simulink model "control_PV"  (R2019b)
settings: Solver=VariableStepAuto  StartTime=0.0  StopTime=500  RelTol=1e-3
undefined symbols (not defined in the file): sgn
libraries: simulink x1
settings Model: Creator=Alejandro  LastModifiedBy=Alejandro
settings SolverCC: ZeroCrossAlgorithm=Adaptive
settings DebuggingCC: IgnoredZcDiagnostic=none

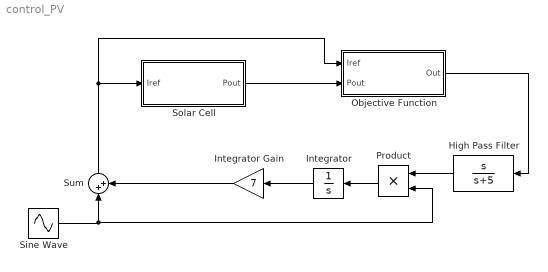
== system control_PV ==
  High Pass Filter : TransferFcn  Numerator=[1 0]  Denominator=[1 5]
  Integrator : Integrator
  Integrator Gain : Gain  Gain=7
  Objective Function : Subsystem  TreatAsAtomicUnit=on
  Product : Product
  Sine Wave : Sin  Amplitude=0.05  Frequency=5*2*pi  SampleTime=0
  Solar Cell : Subsystem
  Sum : Sum  Inputs=|++
  wires:
  High Pass Filter/1 -> Product/1
  Sine Wave/1 -> Product/2, Sum/1
  Product/1 -> Integrator/1
  Integrator/1 -> Integrator Gain/1
  Integrator Gain/1 -> Sum/2
  Objective Function/1(Out) -> High Pass Filter/1
  Solar Cell/1("Pout ") -> Objective Function/2(Pout)
  Sum/1 -> Objective Function/1(Iref), Solar Cell/1("Iref ")

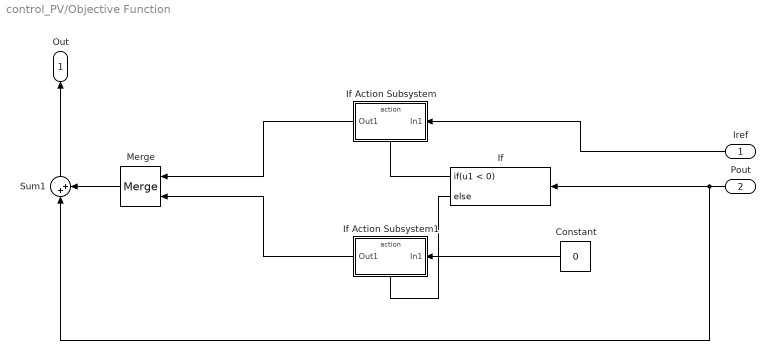
== system control_PV/Objective Function ==
  Iref : Inport
  Pout : Inport  Port=2
  Constant : Constant  Value=0
  If : If  IfExpression=u1 < 0
  If Action Subsystem : Subsystem  TreatAsAtomicUnit=on
  If Action Subsystem1 : Subsystem  TreatAsAtomicUnit=on
  Merge : Merge
  Sum1 : Sum  Inputs=|++
  Out : Outport
  wires:
  If Action Subsystem1/1(Out1) -> Merge/2
  Constant/1 -> If Action Subsystem1/1(In1)
  If/2 -> If Action Subsystem1/Action
  If Action Subsystem/1(Out1) -> Merge/1
  If/1 -> If Action Subsystem/Action
  Iref/1 -> If Action Subsystem/1(In1)
  Merge/1 -> Sum1/2
  Pout/1 -> Sum1/1, If/1
  Sum1/1 -> Out/1

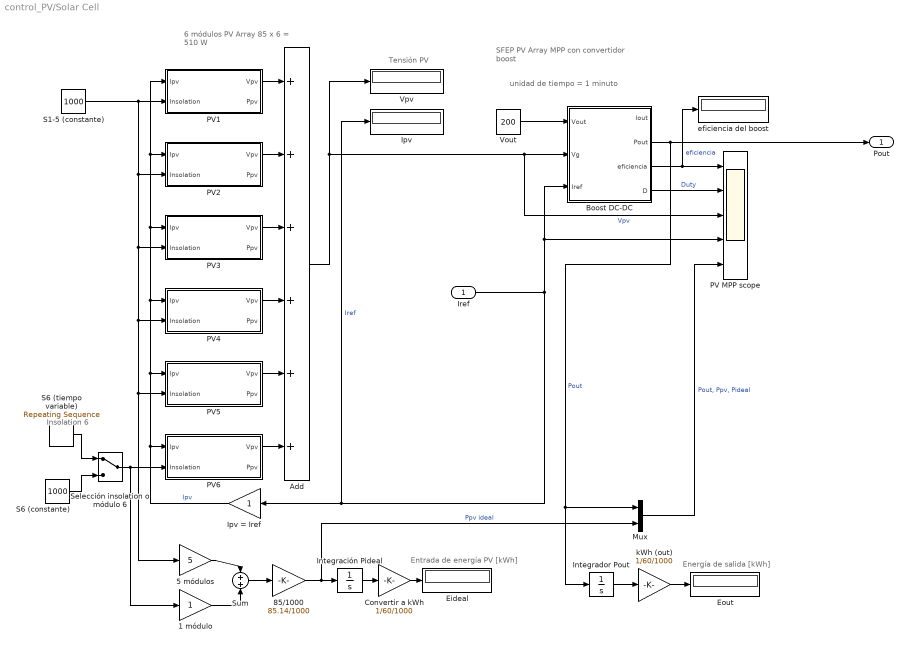
== system control_PV/Solar Cell ==
  note: 6 módulos PV Array
      | 85 x 6 = 510 W
  note: Insolation 6
  note: unidad de tiempo = 1 minuto
  note: SFEP
      | PV Array MPP con convertidor boost
  note: Entrada de energía PV [kWh]
  note: Energía de salida [kWh]
  note: Tensión PV
  "Iref " : Inport
  1 módulo : Gain
  5 módulos : Gain  Gain=5
  85/1000 : Gain  Gain=85.14/1000
  Add : Sum  Inputs=++++++
  Boost DC-DC : Subsystem  mask{RL=0.5, Isw=0.03}
      mask prompts: RL "Resistencia de pérdidas de conducción RL"; Isw "Pérdidas de conmutación Isw"
      mask help: Modelo promediado del boost con corriente de referencia como variable de control. El modelo incluye las pérdidas por conducción en serie con la entrada y la corriente de pérdidas por conmutación en paralelo con la salida.
      mask Display:
      | text(0.5,0.9,'Boost','horizontalAlignment', 'center');
      | text(0.5,0.8,'DC-DC','horizontalAlignment', 'center');
      | text(0.5,0.7,'(control Iref)','horizontalAlignment', 'center');
      | text(0.5,0.6,'promediado','horizontalAlignment', 'center');
  Convertir a kWh : Gain  Gain=1/60/1000
  Eideal : Display
  Eout : Display
  Integración Pideal : Integrator
  Integrador Pout : Integrator
  Ipv : Display
  Ipv = Iref : Gain
  Mux : Mux  Inputs=3
  PV MPP scope : Scope  NumInputPorts=5
  PV1 : Subsystem  mask{Isc=5.45, Voc=22.2, Ir=4.95, Vr=17.2}
      mask prompts: Isc "Corriente de cortocircuito"; Voc "Tensión en circuito abierto"; Ir "Corriente a Pmax"; Vr "Tensión a Pmáx"
      mask help: Modelo de módulo PV. Este modelo tiene entrada de Vpv para realizar conexión en paralelo.
      mask init:
      | % cálculo de PV parámetros
      | % limitación: constante de temperatura
      | Ns = round(Voc/0.61); % por defecto, número de células en serie
      | Vt = 26e-3; % tensión de temperatura
      | G = Isc/1000; % Ganancia de irradiación en función del cortocircuito
      | Vmpc = Vr/Ns; % tensión de celda a Pmáx
      | Vocc = Voc/Ns; % tensión de celda a circuito abierto
      | Rmpp = Vmpc/Ir; % resistencia de carga 
      | %
      | Rp = 100*Vocc/Isc; % valor inicial de Rp
      | Vdm = Vocc; % valor inicial para Vm
      | %
      | % solución iterativa para el modelo: Io, Rs, Rp
      | for i=1:10
      | %
      |  Idm = Isc - Ir - Vdm/Rp; % pn-junction (diodo) corriente a MPP
      |  Io = (Isc-Vocc/Rp)/(exp(Vocc/Vt)-1); % pn-junction corriente inversa de saturación
      |  Vdm = Vt*log(Idm/Io+1); % pn-junction (diodo) tensión a MPP
      |  Rs = (Vdm-Vmpc)/Ir; % resistencia serie
      |  Rd = (Rmpp - Rs)*Rp/(Rp-Rmpp+Rs); % resistencia incremental del diodo  a MPP
      |  Idm = Vt/Rd; % corriente del diodo a MPP basado en resistencia incremental
      |  Rp = Vdm/(Isc-Ir-Idm); % resistencia paralelo
      | %
      | end
      | %
      mask Display:
      | plot([0.3 0.4],[0.4 0.8]);
      | plot([0.4 0.5],[0.4 0.8]);
      | plot([0.5 0.6],[0.4 0.8]);
      | plot([0.6 0.7],[0.4 0.8]);
      | plot([0.3 0.6],[0.4 0.4]);
      | plot([0.325 0.625],[0.5 0.5]);
      | plot([0.35 0.65],[0.6 0.6]);
      | plot([0.375 0.675],[0.7 0.7]);
      | plot([0.4 0.7],[0.8 0.8]);
      | text(0.5,0.9,'Módulo PV','horizontalAlignment', 'center');
  PV2 : Subsystem  mask{Isc=5.45, Voc=22.2, Ir=4.95, Vr=17.2}
      mask prompts: Isc "Corriente de cortocircuito"; Voc "Tensión en circuito abierto"; Ir "Corriente a Pmax"; Vr "Tensión a Pmáx"
      mask help: Modelo de módulo PV. Este modelo tiene entrada de Vpv para realizar conexión en paralelo.
      mask init: same as control_PV/Solar Cell/PV1
      mask Display:
      | plot([0.3 0.4],[0.4 0.8]);
      | plot([0.4 0.5],[0.4 0.8]);
      | plot([0.5 0.6],[0.4 0.8]);
      | plot([0.6 0.7],[0.4 0.8]);
      | plot([0.3 0.6],[0.4 0.4]);
      | plot([0.325 0.625],[0.5 0.5]);
      | plot([0.35 0.65],[0.6 0.6]);
      | plot([0.375 0.675],[0.7 0.7]);
      | plot([0.4 0.7],[0.8 0.8]);
      | text(0.5,0.9,'Módulo PV','horizontalAlignment', 'center');
  PV3 : Subsystem  mask{Isc=5.45, Voc=22.2, Ir=4.95, Vr=17.2}
      mask prompts: Isc "Corriente de cortocircuito"; Voc "Tensión en circuito abierto"; Ir "Corriente a Pmax"; Vr "Tensión a Pmáx"
      mask help: Modelo de módulo PV. Este modelo tiene entrada de Vpv para realizar conexión en paralelo.
      mask init: same as control_PV/Solar Cell/PV1
      mask Display:
      | plot([0.3 0.4],[0.4 0.8]);
      | plot([0.4 0.5],[0.4 0.8]);
      | plot([0.5 0.6],[0.4 0.8]);
      | plot([0.6 0.7],[0.4 0.8]);
      | plot([0.3 0.6],[0.4 0.4]);
      | plot([0.325 0.625],[0.5 0.5]);
      | plot([0.35 0.65],[0.6 0.6]);
      | plot([0.375 0.675],[0.7 0.7]);
      | plot([0.4 0.7],[0.8 0.8]);
      | text(0.5,0.9,'Módulo PV','horizontalAlignment', 'center');
  PV4 : Subsystem  mask{Isc=5.45, Voc=22.2, Ir=4.95, Vr=17.2}
      mask prompts: Isc "Corriente de cortocircuito"; Voc "Tensión en circuito abierto"; Ir "Corriente a Pmax"; Vr "Tensión a Pmáx"
      mask help: Modelo de módulo PV. Este modelo tiene entrada de Vpv para realizar conexión en paralelo.
      mask init: same as control_PV/Solar Cell/PV1
      mask Display:
      | plot([0.3 0.4],[0.4 0.8]);
      | plot([0.4 0.5],[0.4 0.8]);
      | plot([0.5 0.6],[0.4 0.8]);
      | plot([0.6 0.7],[0.4 0.8]);
      | plot([0.3 0.6],[0.4 0.4]);
      | plot([0.325 0.625],[0.5 0.5]);
      | plot([0.35 0.65],[0.6 0.6]);
      | plot([0.375 0.675],[0.7 0.7]);
      | plot([0.4 0.7],[0.8 0.8]);
      | text(0.5,0.9,'Módulo PV','horizontalAlignment', 'center');
  PV5 : Subsystem  mask{Isc=5.45, Voc=22.2, Ir=4.95, Vr=17.2}
      mask prompts: Isc "Corriente de cortocircuito"; Voc "Tensión en circuito abierto"; Ir "Corriente a Pmax"; Vr "Tensión a Pmáx"
      mask help: Modelo de módulo PV. Este modelo tiene entrada de Vpv para realizar conexión en paralelo.
      mask init: same as control_PV/Solar Cell/PV1
      mask Display:
      | plot([0.3 0.4],[0.4 0.8]);
      | plot([0.4 0.5],[0.4 0.8]);
      | plot([0.5 0.6],[0.4 0.8]);
      | plot([0.6 0.7],[0.4 0.8]);
      | plot([0.3 0.6],[0.4 0.4]);
      | plot([0.325 0.625],[0.5 0.5]);
      | plot([0.35 0.65],[0.6 0.6]);
      | plot([0.375 0.675],[0.7 0.7]);
      | plot([0.4 0.7],[0.8 0.8]);
      | text(0.5,0.9,'Módulo PV','horizontalAlignment', 'center');
  PV6 : Subsystem  mask{Isc=5.45, Voc=22.2, Ir=4.95, Vr=17.2}
      mask prompts: Isc "Corriente de cortocircuito"; Voc "Tensión en circuito abierto"; Ir "Corriente a Pmax"; Vr "Tensión a Pmáx"
      mask help: Modelo de módulo PV. Este modelo tiene entrada de Vpv para realizar conexión en paralelo.
      mask init: same as control_PV/Solar Cell/PV1
      mask Display:
      | plot([0.3 0.4],[0.4 0.8]);
      | plot([0.4 0.5],[0.4 0.8]);
      | plot([0.5 0.6],[0.4 0.8]);
      | plot([0.6 0.7],[0.4 0.8]);
      | plot([0.3 0.6],[0.4 0.4]);
      | plot([0.325 0.625],[0.5 0.5]);
      | plot([0.35 0.65],[0.6 0.6]);
      | plot([0.375 0.675],[0.7 0.7]);
      | plot([0.4 0.7],[0.8 0.8]);
      | text(0.5,0.9,'Módulo PV','horizontalAlignment', 'center');
  S1-5 (constante) : Constant  Value=1000
  S6 (tiempo variable) : simulink/Sources/Repeating Sequence  rep_seq_t=[0 1*60 2*60 3*60 4*60 5*60 6*60 7*60 8*60]  rep_seq_y=[0 400 850 950 0 950 850 400 0]
  S6 (constante) : Constant  Value=1000
  Selección insolation o módulo 6 : ManualSwitch
  Sum : Sum  Inputs=+|+
  Vout : Constant  Value=200
  Vpv : Display
  eficiencia del boost : Display
  kWh (out) : Gain  Gain=1/60/1000
  "Pout " : Outport
  wires:
  PV1/1(Vpv) -> Add/1
  Ipv = Iref/1 -> PV2/1(Ipv), PV1/1(Ipv), PV3/1(Ipv), PV4/1(Ipv), PV5/1(Ipv), PV6/1(Ipv)  "Ipv"
  PV2/1(Vpv) -> Add/2
  Boost DC-DC/2(Pout) -> "Pout "/1, Mux/1, Integrador Pout/1  "Pout"
  S6 (tiempo variable)/1 -> Selección insolation o módulo 6/1
  kWh (out)/1 -> Eout/1
  "Iref "/1 -> Ipv = Iref/1, Ipv/1, Boost DC-DC/3(Iref), PV MPP scope/4  "Iref"
  PV6/1(Vpv) -> Add/6
  Boost DC-DC/3(eficiencia) -> eficiencia del boost/1, PV MPP scope/1  "eficiencia"
  Selección insolation o módulo 6/1 -> 1 módulo/1, PV6/2(Insolation)
  Convertir a kWh/1 -> Eideal/1
  Integrador Pout/1 -> kWh (out)/1
  PV4/1(Vpv) -> Add/4
  Vout/1 -> Boost DC-DC/1(Vout)
  Add/1 -> Vpv/1, Boost DC-DC/2(Vg), PV MPP scope/3  "Vpv"
  Boost DC-DC/4(D) -> PV MPP scope/2  "Duty"
  5 módulos/1 -> Sum/1
  Sum/1 -> 85/1000/1
  PV3/1(Vpv) -> Add/3
  1 módulo/1 -> Sum/2
  85/1000/1 -> Integración Pideal/1, Mux/3  "Ppv ideal"
  Mux/1 -> PV MPP scope/5  "Pout, Ppv, Pideal"
  S1-5 (constante)/1 -> 5 módulos/1, PV5/2(Insolation), PV4/2(Insolation), PV3/2(Insolation), PV2/2(Insolation), PV1/2(Insolation)
  PV5/1(Vpv) -> Add/5
  S6 (constante)/1 -> Selección insolation o módulo 6/2
  Integración Pideal/1 -> Convertir a kWh/1

== system control_PV/Objective Function/If Action Subsystem ==
  In1 : Inport
  Action Port : ActionPort  ActionPortLabel=if(u1 < 0)
  Fcn : Fcn  Expr=-sgn(u)*u*5-6
  Out1 : Outport
  wires:
  In1/1 -> Fcn/1
  Fcn/1 -> Out1/1

== system control_PV/Objective Function/If Action Subsystem1 ==
  In1 : Inport
  Action Port : ActionPort  ActionPortLabel=else
  Out1 : Outport
  wires:
  In1/1 -> Out1/1

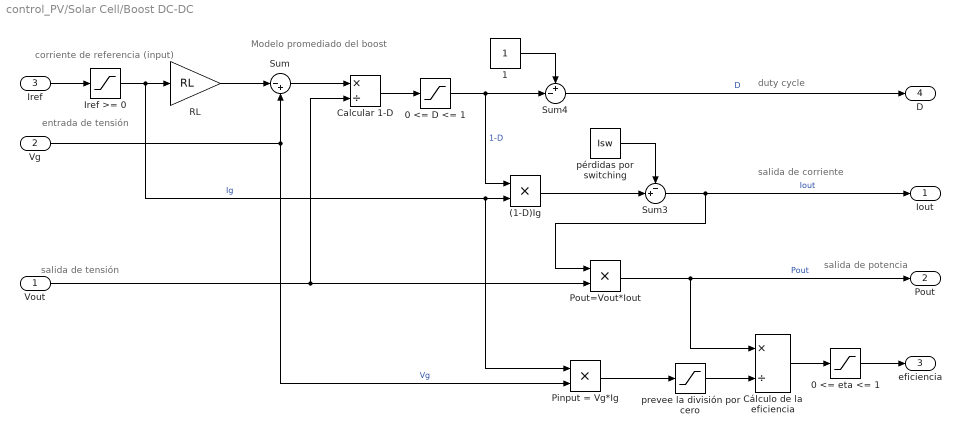
== system control_PV/Solar Cell/Boost DC-DC ==
  note: Modelo promediado del boost
  note: salida de corriente
  note: salida de tensión
  note: entrada de tensión
  note: corriente de
      | referencia (input)
  note: duty cycle
  note: salida de potencia
  Vout : Inport
  Vg : Inport  Port=2
  Iref : Inport  Port=3
  (1-D)Ig : Product  Inputs=**  RndMeth=Zero
  0 <= D <= 1 : Saturate  UpperLimit=1  LowerLimit=0
  0 <= eta <= 1 : Saturate  UpperLimit=1  LowerLimit=0
  1 : Constant
  Calcular 1-D : Product  Inputs=*/  RndMeth=Zero
  Cálculo de la eficiencia : Product  Inputs=*/  RndMeth=Zero
  Iref >= 0 : Saturate  UpperLimit=inf  LowerLimit=0
  Pinput = Vg*Ig : Product  Inputs=**  RndMeth=Zero
  Pout=Vout*Iout : Product  Inputs=**  RndMeth=Zero
  RL : Gain  Gain=RL
  Sum : Sum  Inputs=|-+
  Sum3 : Sum  Inputs=-+|
  Sum4 : Sum  Inputs=+-|
  prevee la división por cero : Saturate  UpperLimit=inf  LowerLimit=eps
  pérdidas por switching : Constant  Value=Isw
  Iout : Outport
  Pout : Outport  Port=2
  eficiencia : Outport  Port=3
  D : Outport  Port=4
  wires:
  Cálculo de la eficiencia/1 -> 0 <= eta <= 1/1
  Iref/1 -> Iref >= 0/1
  Vout/1 -> Pout=Vout*Iout/2, Calcular 1-D/2
  pérdidas por switching/1 -> Sum3/1
  Sum3/1 -> Iout/1, Pout=Vout*Iout/1  "Iout"
  Pout=Vout*Iout/1 -> Pout/1, Cálculo de la eficiencia/1  "Pout"
  0 <= eta <= 1/1 -> eficiencia/1
  Iref >= 0/1 -> RL/1, (1-D)Ig/2, Pinput = Vg*Ig/1  "Ig"
  RL/1 -> Sum/1
  Vg/1 -> Sum/2, Pinput = Vg*Ig/2  "Vg"
  Sum/1 -> Calcular 1-D/1
  Calcular 1-D/1 -> 0 <= D <= 1/1
  0 <= D <= 1/1 -> Sum4/2, (1-D)Ig/1  "1-D"
  1/1 -> Sum4/1
  Sum4/1 -> D/1  "D"
  (1-D)Ig/1 -> Sum3/2
  prevee la división por cero/1 -> Cálculo de la eficiencia/2
  Pinput = Vg*Ig/1 -> prevee la división por cero/1

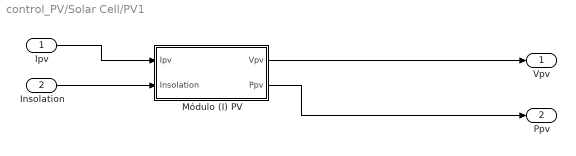
== system control_PV/Solar Cell/PV1 ==
  Ipv : Inport
  Insolation : Inport  Port=2
  Módulo (I) PV : Subsystem
  Vpv : Outport
  Ppv : Outport  Port=2
  wires:
  Insolation/1 -> Módulo (I) PV/2(Insolation)
  Módulo (I) PV/2(Ppv) -> Ppv/1
  Ipv/1 -> Módulo (I) PV/1(Ipv)
  Módulo (I) PV/1(Vpv) -> Vpv/1

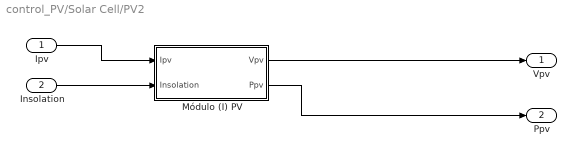
== system control_PV/Solar Cell/PV2 ==
  Ipv : Inport
  Insolation : Inport  Port=2
  Módulo (I) PV : Subsystem
  Vpv : Outport
  Ppv : Outport  Port=2
  wires:
  Insolation/1 -> Módulo (I) PV/2(Insolation)
  Módulo (I) PV/2(Ppv) -> Ppv/1
  Ipv/1 -> Módulo (I) PV/1(Ipv)
  Módulo (I) PV/1(Vpv) -> Vpv/1

== system control_PV/Solar Cell/PV3 ==
  Ipv : Inport
  Insolation : Inport  Port=2
  Módulo (I) PV : Subsystem
  Vpv : Outport
  Ppv : Outport  Port=2
  wires:
  Insolation/1 -> Módulo (I) PV/2(Insolation)
  Módulo (I) PV/2(Ppv) -> Ppv/1
  Ipv/1 -> Módulo (I) PV/1(Ipv)
  Módulo (I) PV/1(Vpv) -> Vpv/1

== system control_PV/Solar Cell/PV4 ==
  Ipv : Inport
  Insolation : Inport  Port=2
  Módulo (I) PV : Subsystem
  Vpv : Outport
  Ppv : Outport  Port=2
  wires:
  Insolation/1 -> Módulo (I) PV/2(Insolation)
  Módulo (I) PV/2(Ppv) -> Ppv/1
  Ipv/1 -> Módulo (I) PV/1(Ipv)
  Módulo (I) PV/1(Vpv) -> Vpv/1

== system control_PV/Solar Cell/PV5 ==
  Ipv : Inport
  Insolation : Inport  Port=2
  Módulo (I) PV : Subsystem
  Vpv : Outport
  Ppv : Outport  Port=2
  wires:
  Insolation/1 -> Módulo (I) PV/2(Insolation)
  Módulo (I) PV/2(Ppv) -> Ppv/1
  Ipv/1 -> Módulo (I) PV/1(Ipv)
  Módulo (I) PV/1(Vpv) -> Vpv/1

== system control_PV/Solar Cell/PV6 ==
  Ipv : Inport
  Insolation : Inport  Port=2
  Módulo (I) PV : Subsystem
  Vpv : Outport
  Ppv : Outport  Port=2
  wires:
  Insolation/1 -> Módulo (I) PV/2(Insolation)
  Módulo (I) PV/2(Ppv) -> Ppv/1
  Ipv/1 -> Módulo (I) PV/1(Ipv)
  Módulo (I) PV/1(Vpv) -> Vpv/1

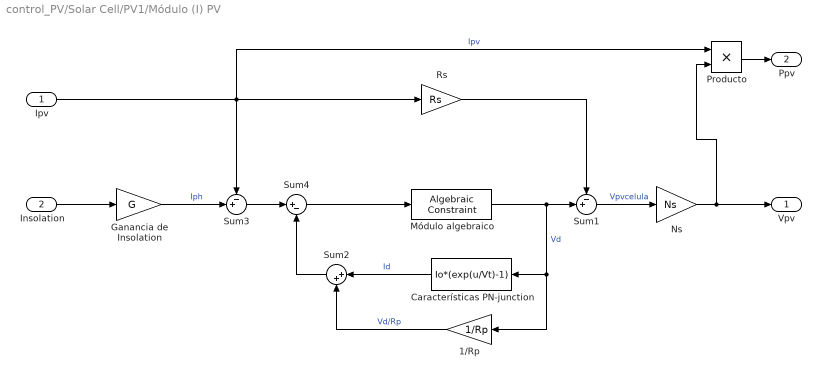
== system control_PV/Solar Cell/PV1/Módulo (I) PV ==
  Ipv : Inport
  Insolation : Inport  Port=2
  1/Rp : Gain  Gain=1/Rp
  Características PN-junction : Fcn  Expr=Io*(exp(u/Vt)-1)
  Ganancia de Insolation : Gain  Gain=G
  Módulo algebraico : AlgebraicConstraint
  Ns : Gain  Gain=Ns
  Producto : Product  RndMeth=Zero
  Rs : Gain  Gain=Rs
  Sum1 : Sum  Inputs=-+|
  Sum2 : Sum  Inputs=|++
  Sum3 : Sum  Inputs=-+|
  Sum4 : Sum  Inputs=|+-
  Vpv : Outport
  Ppv : Outport  Port=2
  wires:
  Insolation/1 -> Ganancia de Insolation/1
  Ganancia de Insolation/1 -> Sum3/2  "Iph"
  Ipv/1 -> Sum3/1, Rs/1, Producto/1  "Ipv"
  Producto/1 -> Ppv/1
  Sum4/1 -> Módulo algebraico/1
  Módulo algebraico/1 -> Sum1/2, 1/Rp/1, Características PN-junction/1  "Vd"
  Sum1/1 -> Ns/1  "Vpvcelula"
  Rs/1 -> Sum1/1
  Sum3/1 -> Sum4/1
  Sum2/1 -> Sum4/2
  Características PN-junction/1 -> Sum2/1  "Id"
  1/Rp/1 -> Sum2/2  "Vd/Rp"
  Ns/1 -> Vpv/1, Producto/2

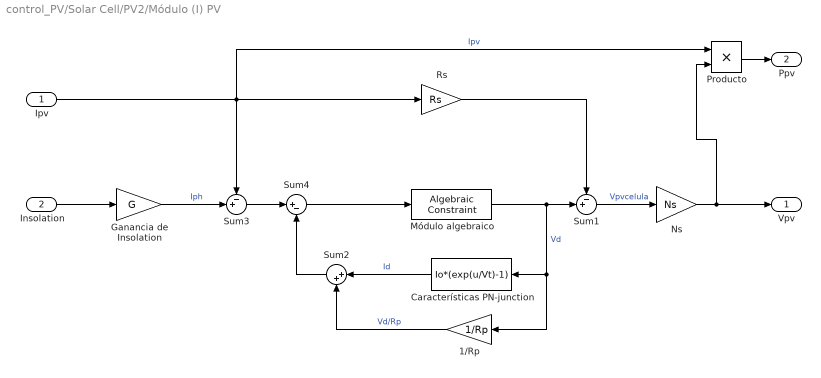
== system control_PV/Solar Cell/PV2/Módulo (I) PV ==
  Ipv : Inport
  Insolation : Inport  Port=2
  1/Rp : Gain  Gain=1/Rp
  Características PN-junction : Fcn  Expr=Io*(exp(u/Vt)-1)
  Ganancia de Insolation : Gain  Gain=G
  Módulo algebraico : AlgebraicConstraint
  Ns : Gain  Gain=Ns
  Producto : Product  RndMeth=Zero
  Rs : Gain  Gain=Rs
  Sum1 : Sum  Inputs=-+|
  Sum2 : Sum  Inputs=|++
  Sum3 : Sum  Inputs=-+|
  Sum4 : Sum  Inputs=|+-
  Vpv : Outport
  Ppv : Outport  Port=2
  wires:
  Insolation/1 -> Ganancia de Insolation/1
  Ganancia de Insolation/1 -> Sum3/2  "Iph"
  Ipv/1 -> Sum3/1, Rs/1, Producto/1  "Ipv"
  Producto/1 -> Ppv/1
  Sum4/1 -> Módulo algebraico/1
  Módulo algebraico/1 -> Sum1/2, 1/Rp/1, Características PN-junction/1  "Vd"
  Sum1/1 -> Ns/1  "Vpvcelula"
  Rs/1 -> Sum1/1
  Sum3/1 -> Sum4/1
  Sum2/1 -> Sum4/2
  Características PN-junction/1 -> Sum2/1  "Id"
  1/Rp/1 -> Sum2/2  "Vd/Rp"
  Ns/1 -> Vpv/1, Producto/2

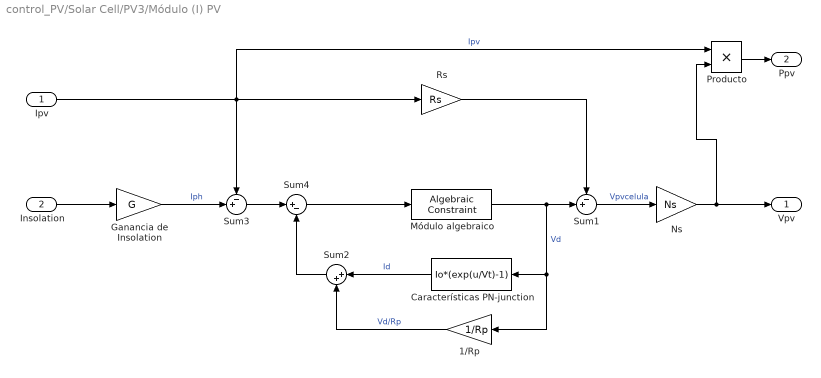
== system control_PV/Solar Cell/PV3/Módulo (I) PV ==
  Ipv : Inport
  Insolation : Inport  Port=2
  1/Rp : Gain  Gain=1/Rp
  Características PN-junction : Fcn  Expr=Io*(exp(u/Vt)-1)
  Ganancia de Insolation : Gain  Gain=G
  Módulo algebraico : AlgebraicConstraint
  Ns : Gain  Gain=Ns
  Producto : Product  RndMeth=Zero
  Rs : Gain  Gain=Rs
  Sum1 : Sum  Inputs=-+|
  Sum2 : Sum  Inputs=|++
  Sum3 : Sum  Inputs=-+|
  Sum4 : Sum  Inputs=|+-
  Vpv : Outport
  Ppv : Outport  Port=2
  wires:
  Insolation/1 -> Ganancia de Insolation/1
  Ganancia de Insolation/1 -> Sum3/2  "Iph"
  Ipv/1 -> Sum3/1, Rs/1, Producto/1  "Ipv"
  Producto/1 -> Ppv/1
  Sum4/1 -> Módulo algebraico/1
  Módulo algebraico/1 -> Sum1/2, 1/Rp/1, Características PN-junction/1  "Vd"
  Sum1/1 -> Ns/1  "Vpvcelula"
  Rs/1 -> Sum1/1
  Sum3/1 -> Sum4/1
  Sum2/1 -> Sum4/2
  Características PN-junction/1 -> Sum2/1  "Id"
  1/Rp/1 -> Sum2/2  "Vd/Rp"
  Ns/1 -> Vpv/1, Producto/2

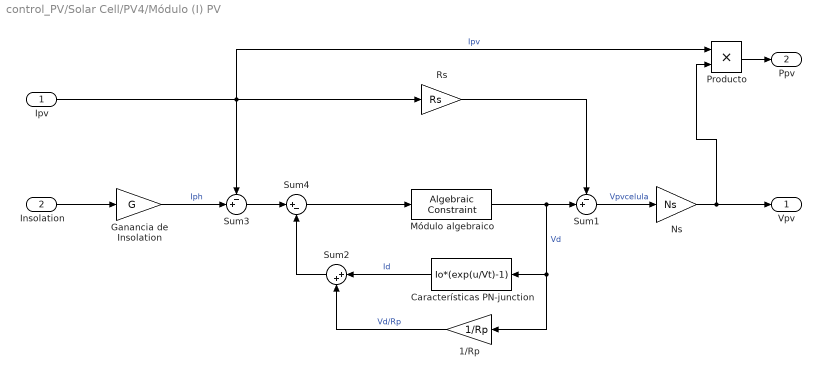
== system control_PV/Solar Cell/PV4/Módulo (I) PV ==
  Ipv : Inport
  Insolation : Inport  Port=2
  1/Rp : Gain  Gain=1/Rp
  Características PN-junction : Fcn  Expr=Io*(exp(u/Vt)-1)
  Ganancia de Insolation : Gain  Gain=G
  Módulo algebraico : AlgebraicConstraint
  Ns : Gain  Gain=Ns
  Producto : Product  RndMeth=Zero
  Rs : Gain  Gain=Rs
  Sum1 : Sum  Inputs=-+|
  Sum2 : Sum  Inputs=|++
  Sum3 : Sum  Inputs=-+|
  Sum4 : Sum  Inputs=|+-
  Vpv : Outport
  Ppv : Outport  Port=2
  wires:
  Insolation/1 -> Ganancia de Insolation/1
  Ganancia de Insolation/1 -> Sum3/2  "Iph"
  Ipv/1 -> Sum3/1, Rs/1, Producto/1  "Ipv"
  Producto/1 -> Ppv/1
  Sum4/1 -> Módulo algebraico/1
  Módulo algebraico/1 -> Sum1/2, 1/Rp/1, Características PN-junction/1  "Vd"
  Sum1/1 -> Ns/1  "Vpvcelula"
  Rs/1 -> Sum1/1
  Sum3/1 -> Sum4/1
  Sum2/1 -> Sum4/2
  Características PN-junction/1 -> Sum2/1  "Id"
  1/Rp/1 -> Sum2/2  "Vd/Rp"
  Ns/1 -> Vpv/1, Producto/2

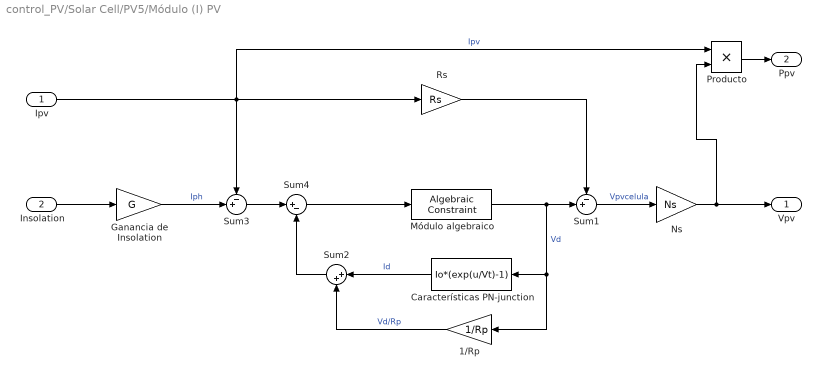
== system control_PV/Solar Cell/PV5/Módulo (I) PV ==
  Ipv : Inport
  Insolation : Inport  Port=2
  1/Rp : Gain  Gain=1/Rp
  Características PN-junction : Fcn  Expr=Io*(exp(u/Vt)-1)
  Ganancia de Insolation : Gain  Gain=G
  Módulo algebraico : AlgebraicConstraint
  Ns : Gain  Gain=Ns
  Producto : Product  RndMeth=Zero
  Rs : Gain  Gain=Rs
  Sum1 : Sum  Inputs=-+|
  Sum2 : Sum  Inputs=|++
  Sum3 : Sum  Inputs=-+|
  Sum4 : Sum  Inputs=|+-
  Vpv : Outport
  Ppv : Outport  Port=2
  wires:
  Insolation/1 -> Ganancia de Insolation/1
  Ganancia de Insolation/1 -> Sum3/2  "Iph"
  Ipv/1 -> Sum3/1, Rs/1, Producto/1  "Ipv"
  Producto/1 -> Ppv/1
  Sum4/1 -> Módulo algebraico/1
  Módulo algebraico/1 -> Sum1/2, 1/Rp/1, Características PN-junction/1  "Vd"
  Sum1/1 -> Ns/1  "Vpvcelula"
  Rs/1 -> Sum1/1
  Sum3/1 -> Sum4/1
  Sum2/1 -> Sum4/2
  Características PN-junction/1 -> Sum2/1  "Id"
  1/Rp/1 -> Sum2/2  "Vd/Rp"
  Ns/1 -> Vpv/1, Producto/2

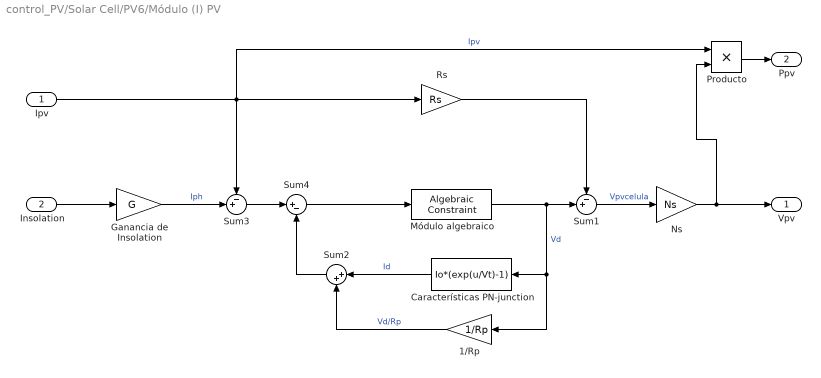
== system control_PV/Solar Cell/PV6/Módulo (I) PV ==
  Ipv : Inport
  Insolation : Inport  Port=2
  1/Rp : Gain  Gain=1/Rp
  Características PN-junction : Fcn  Expr=Io*(exp(u/Vt)-1)
  Ganancia de Insolation : Gain  Gain=G
  Módulo algebraico : AlgebraicConstraint
  Ns : Gain  Gain=Ns
  Producto : Product  RndMeth=Zero
  Rs : Gain  Gain=Rs
  Sum1 : Sum  Inputs=-+|
  Sum2 : Sum  Inputs=|++
  Sum3 : Sum  Inputs=-+|
  Sum4 : Sum  Inputs=|+-
  Vpv : Outport
  Ppv : Outport  Port=2
  wires:
  Insolation/1 -> Ganancia de Insolation/1
  Ganancia de Insolation/1 -> Sum3/2  "Iph"
  Ipv/1 -> Sum3/1, Rs/1, Producto/1  "Ipv"
  Producto/1 -> Ppv/1
  Sum4/1 -> Módulo algebraico/1
  Módulo algebraico/1 -> Sum1/2, 1/Rp/1, Características PN-junction/1  "Vd"
  Sum1/1 -> Ns/1  "Vpvcelula"
  Rs/1 -> Sum1/1
  Sum3/1 -> Sum4/1
  Sum2/1 -> Sum4/2
  Características PN-junction/1 -> Sum2/1  "Id"
  1/Rp/1 -> Sum2/2  "Vd/Rp"
  Ns/1 -> Vpv/1, Producto/2
